simulink model "Control_model_10DOF_fin"  (R2016b)
settings: Solver=FixedStepAuto  StartTime=0.0  StopTime=10  FixedStep=0.0001  RelTol=1e-3
InitFcn:
  | Initialisation_ctr_10DOF_fin
values from neighbouring files (symbols this model uses):
  COM_Parameters = [-lpelvis/2;r2;0]    [Initialisation_ctr_10DOF_fin.m]
  DH_Parameters = [hfoot 0 ... (first row only)    [Initialisation_ctr_10DOF_fin.m]
  dTrunk = trunklbd(3)    [Initialisation_ctr_10DOF_fin.m]
  dxFootSM = dxFoot    [Initialisation_ctr_10DOF_fin.m]
  dxTrunk = 0.1    [Initialisation_ctr_10DOF_fin.m]
  Foot_Parameters = [0;-(lFoot/2-lHeel);0]    [Initialisation_ctr_10DOF_fin.m]
  HAA2HEE = [0; 0; 0.001]    [Initialisation_ctr_10DOF_fin.m]
  HEE2HFE = 0.5*[0.2; 0; 0]    [Initialisation_ctr_10DOF_fin.m]
  height_vrp = CoM_position(1)    [Initialisation_ctr_10DOF_fin.m]
  hTrunk = trunklbd(1)    [Initialisation_ctr_10DOF_fin.m]
  initial_CoM_position = R*CoM_position    [Initialisation_ctr_10DOF_fin.m]
  initial_CoM_velocity = [0;0;0]    [Initialisation_ctr_10DOF_fin.m]
  initial_left_foot = [0;0;-stance_width/2]    [Initialisation_ctr_10DOF_fin.m]
  initial_right_foot = [0;0;stance_width/2]    [Initialisation_ctr_10DOF_fin.m]
  initial_RorL = 0    [Initialisation_ctr_10DOF_fin.m]
  jointsinitial = [9;-15;6;0;0;6;-15;9]/180*pi    [Initialisation_ctr_10DOF_fin.m]
  K_DCM = 4.3*[1 0 0 ... (first row only)    [Initialisation_ctr_10DOF_fin.m]
  kD_left = mbody*[0.95 0 0 0 ... (first row only)    [Initialisation_ctr_10DOF_fin.m]
  kD_right = mbody*[0.12 0 0 0 ... (first row only)    [Initialisation_ctr_10DOF_fin.m]
  kI_left = mbody*[35 0 0 0 ... (first row only)    [Initialisation_ctr_10DOF_fin.m]
  kI_right = mbody*[38.2 0 0 0 ... (first row only)    [Initialisation_ctr_10DOF_fin.m]
  kP_left = mbody*[75 0 0 0 ... (first row only)    [Initialisation_ctr_10DOF_fin.m]
  kP_right = mbody*[5.6 0 0 0 ... (first row only)    [Initialisation_ctr_10DOF_fin.m]
  Lenght = [lShank;lThigh]    [Initialisation_ctr_10DOF_fin.m]
  lFootSM = lFoot    [Initialisation_ctr_10DOF_fin.m]
  lpelvis = wPelvis    [Initialisation_ctr_10DOF_fin.m]
  mass = mbody    (= 60)    [Initialisation_ctr_10DOF_fin.m]
  Masses = [mThigh; mShank; mTrunk]    [Initialisation_ctr_10DOF_fin.m]
  nb_step = 4    [Initialisation_ctr_10DOF_fin.m]
  nb_step_pattern = 20    [Initialisation_ctr_10DOF_fin.m]
  Pelvis_Parameters = [-lpelvis/2;hTrunk/2;0]    [Initialisation_ctr_10DOF_fin.m]
  stance_width = lpelvis    [Initialisation_ctr_10DOF_fin.m]
  stride_lenght = 0.50    (= 0.5)    [Initialisation_ctr_10DOF_fin.m]
  T_DS = time_DS    (= 0.4)    [Initialisation_ctr_10DOF_fin.m]
  T_IT = time_DS    (= 0.4)    [Initialisation_ctr_10DOF_fin.m]
  T_SS = time_swing    (= 1.6)    [Initialisation_ctr_10DOF_fin.m]
  time_DS = (time_stance-time_swing)/2    (= 0.4)    [Initialisation_ctr_10DOF_fin.m]
  time_stance = 60/100*time_stride    (= 2.4)    [Initialisation_ctr_10DOF_fin.m]
  time_step = time_stride/2    (= 2)    [Initialisation_ctr_10DOF_fin.m]
  time_swing = 40/100*time_stride    (= 1.6)    [Initialisation_ctr_10DOF_fin.m]
  validity_angle = [-20*pi/180 20*pi/180 ... (first row only)    [Initialisation_ctr_10DOF_fin.m]
  wTrunk = trunklbd(2)    [Initialisation_ctr_10DOF_fin.m]
  x4CoM = CoM_position(1)-XR4(1)    [Initialisation_ctr_10DOF_fin.m]
undefined symbols (not defined in the file or in its folder): dsegment, hFoot, l, lFoot, omega0_x, omega0_z, rho, wPelvis, X, Xp_x, Xp_z, Y, Z
undefined symbols (not defined in the file): k_grf, lShankSM, lThighSM, mShank, mThigh
libraries: nesl_utility x247, sm_lib x215, dspindex x12, FootPlacementLibrary x8, dspsigops x4, dspswit3 x1
(part 11 of 18)

== system Control_model_10DOF_fin/Control/Single_Support/Left Swing // Right Stance/Scope x8 ==
  Input : Inport
  Demux : Demux  Outputs=3
  Scope1 : Scope
  Scope2 : Scope
  Scope3 : Scope
  wires:
  Input/1 -> Demux/1
  Demux/2 -> Scope1/1
  Demux/3 -> Scope2/1
  Demux/1 -> Scope3/1

== system Control_model_10DOF_fin/Control/Single_Support/Left Swing // Right Stance/Stance leg position_initial ==
  position : Inport  PortDimensions=4
  velocity : Inport  Port=2  PortDimensions=4
  hip_trajectory : Inport  Port=3
  theta2 : Inport  Port=4
  Constant : Constant  Value=jointsinitial(1:4)
  Demux : Demux
  Mux : Mux
  PID right : Subsystem
  Scope x2 : Subsystem
  Sum1 : Sum  Inputs=-+|
  Terminator : Terminator
  Terminator1 : Terminator
  torques : Outport
  wires:
  PID right/1(torques_des) -> torques/1
  position/1 -> Scope x2/1(Input), Sum1/1
  Sum1/1 -> PID right/1(error)
  velocity/1 -> PID right/2(velocity)
  Constant/1 -> Demux/1
  Mux/1 -> Scope x2/2(Input1), Sum1/2
  Demux/1 -> Mux/1
  Demux/3 -> Mux/3
  hip_trajectory/1 -> Mux/4
  theta2/1 -> Mux/2
  Demux/2 -> Terminator/1
  Demux/4 -> Terminator1/1

== system Control_model_10DOF_fin/Control/Single_Support/Right Swing // Left Stance/Martijn Step adjustement ==
  FK_info : Inport
  R_or_L : Inport  Port=2
  Bus Selector : BusSelector  OutputSignals=XWcom,VWcom
  Constant1 : Constant  Value=time_swing
  Terminator : Terminator
  xCoM pred : Subsystem
  StepPos : Outport
  wires:
  Constant1/1 -> xCoM pred/1(T)
  R_or_L/1 -> xCoM pred/4(R_or_L)
  FK_info/1 -> Bus Selector/1
  Bus Selector/2 -> xCoM pred/3(Vcom)  "<VWcom>"
  Bus Selector/1 -> xCoM pred/2(Xcom)  "<XWcom>"
  xCoM pred/1(StepPos) -> StepPos/1
  xCoM pred/2(xCoMpred) -> Terminator/1

== system Control_model_10DOF_fin/Control/Single_Support/Right Swing // Left Stance/Right Swing leg control ==
  swing_state : Inport
  actual_joint_angle : Inport  Port=2
  FK_info : Inport  Port=3
  actual_joint_velocity : Inport  Port=4
  theta2 : Inport  Port=5
  Bus Selector : BusSelector  OutputSignals=TL4,TL1,TL0,TLR,TWL
  PID right : Subsystem
  Right : MATLAB Function  TreatAsAtomicUnit=on
  Saturation : Saturate  UpperLimit=validity_angle(1:4,2)  LowerLimit=validity_angle(1:4,1)
  Scope x2 : Subsystem
  Scope1 : Scope
  Scope2 : Scope
  Sum : Sum  Inputs=-+|
  Torques_des : Outport  OutDataTypeStr=double  Unit=N*m  PortDimensions=4
  wires:
  Right/1(desired_joint_angle) -> Saturation/1
  Sum/1 -> PID right/1(error)
  actual_joint_angle/1 -> Right/8(actual_joint_angle), Scope x2/1(Input), Sum/1
  FK_info/1 -> Bus Selector/1
  swing_state/1 -> Right/6(swing_state)
  actual_joint_velocity/1 -> PID right/2(velocity)
  PID right/1(torques_des) -> Torques_des/1
  Bus Selector/1 -> Right/1(TL4)  "<TL4>"
  Bus Selector/2 -> Right/2(TL1)  "<TL1>"
  Bus Selector/3 -> Right/3(TL0)  "<TL0>"
  Bus Selector/4 -> Right/4(TLR)  "<TLR>"
  Bus Selector/5 -> Right/5(TWL)  "<TWL>"
  Right/3(cas) -> Scope1/1
  Saturation/1 -> Sum/2, Scope x2/2(Input1)
  Right/2(ok) -> Scope2/1
  theta2/1 -> Right/7(desired_knee_angle)

== system Control_model_10DOF_fin/Control/Single_Support/Right Swing // Left Stance/Stance leg control ==
  DCM_position : Inport
  DCM_velocity : Inport  Port=2
  FK_info : Inport  Port=3
  Bus Selector : BusSelector  OutputSignals=XWcom,VWcom
  Bus Selector1 : BusSelector  OutputSignals=JLcom,TWL
  Bus Selector2 : BusSelector  OutputSignals=TWL
  Bus Selector3 : BusSelector  OutputSignals=XWcom
  DCM calcul : MATLAB Function  TreatAsAtomicUnit=on
  MATLAB Function : MATLAB Function  TreatAsAtomicUnit=on
  MATLAB Function1 : MATLAB Function  TreatAsAtomicUnit=on
  MATLAB Function2 : MATLAB Function  TreatAsAtomicUnit=on
  MATLAB Function5 : MATLAB Function  TreatAsAtomicUnit=on
  Terminator : Terminator
  Terminator1 : Terminator
  VRP based DCM tracking control : MATLAB Function  TreatAsAtomicUnit=on
  Torques_des : Outport  OutDataTypeStr=double  Unit=N*m
  Force_des : Outport  Port=2
  r_vrp : Outport  Port=3
  r_extrapolated_CoM : Outport  Port=4
  wires:
  DCM_position/1 -> VRP based DCM tracking control/3(DCM_position)
  DCM_velocity/1 -> VRP based DCM tracking control/2(DCM_velocity)
  Bus Selector/1 -> DCM calcul/1(CoM_position)  "<XWcom>"
  DCM calcul/1(r_DCM) -> VRP based DCM tracking control/1(r_DCM), r_extrapolated_CoM/1
  MATLAB Function/1(Force_des) -> MATLAB Function2/1(Force_des)
  MATLAB Function2/1(Torques_des) -> Torques_des/1
  Bus Selector/2 -> DCM calcul/2(CoM_velocity)  "<VWcom>"
  Bus Selector1/1 -> MATLAB Function2/2(JcomL)  "<JLcom>"
  MATLAB Function5/1(new_vrp_W) -> MATLAB Function/1(r_vrp)
  VRP based DCM tracking control/1(r_vrp) -> r_vrp/1, MATLAB Function1/1(r_vrp), MATLAB Function5/1(r_vrp_W)
  Bus Selector2/1 -> MATLAB Function1/3(TWL), MATLAB Function5/2(TWL)  "<TWL>"
  Bus Selector3/1 -> MATLAB Function1/2(r_CoM), MATLAB Function/2(r_CoM)  "<XWcom>"
  Bus Selector1/2 -> MATLAB Function2/3(TWL)  "<TWL>"
  FK_info/1 -> Bus Selector1/1, Bus Selector3/1, Bus Selector2/1, Bus Selector/1
  MATLAB Function1/1(Force_des) -> Force_des/1
  MATLAB Function5/2(outside) -> Terminator/1
  MATLAB Function5/3(cas) -> Terminator1/1

== system Control_model_10DOF_fin/Control/Single_Support/Right Swing // Left Stance/Stance leg position_initial1 ==
  position : Inport  PortDimensions=4
  velocity : Inport  Port=2  PortDimensions=4
  hip_trajectory : Inport  Port=3
  theta7 : Inport  Port=4
  Constant : Constant  Value=jointsinitial(5:8)
  Demux1 : Demux
  Mux1 : Mux
  PID left : Subsystem
  Scope : Scope
  Sum1 : Sum  Inputs=-+|
  Terminator : Terminator
  Terminator1 : Terminator
  torques : Outport
  wires:
  position/1 -> Sum1/1
  Sum1/1 -> Scope/1, PID left/1(error)
  velocity/1 -> PID left/2(velocity)
  PID left/1(torques_des) -> torques/1
  Constant/1 -> Demux1/1
  Mux1/1 -> Sum1/2
  Demux1/2 -> Mux1/2
  Demux1/4 -> Mux1/4
  hip_trajectory/1 -> Mux1/1
  theta7/1 -> Mux1/3
  Demux1/1 -> Terminator/1
  Demux1/3 -> Terminator1/1

== system Control_model_10DOF_fin/Control/Stance_position/Stance control/PID left ==
  error : Inport  PortDimensions=4
  velocity : Inport  Port=2
  Filter : Integrator  Commented=on  DisableCoverage=on
  Gain : Gain  Commented=on  Gain=100
  Integrator : Integrator
  Product{,1..3} (4 alike) : Product  Multiplication=Matrix(*)
  Sum : Sum  Inputs=++-
  Sum1 : Sum  Commented=on  Inputs=|+-
  kD : Constant  Value=kD_left
  kI : Constant  Value=kI_left
  kP : Constant  Value=kP_left
  torques_des : Outport  PortDimensions=4  InitialOutput=0
  wires:
  Sum/1 -> torques_des/1
  Gain/1 -> Filter/1
  Sum1/1 -> Gain/1
  Product/1 -> Sum/1
  error/1 -> Product2/2, Product1/2, Product/2
  Product1/1 -> Sum1/1
  kP/1 -> Product/1
  Filter/1 -> Sum1/2
  Integrator/1 -> Sum/2
  Product2/1 -> Integrator/1
  kI/1 -> Product2/1
  kD/1 -> Product3/1, Product1/1
  velocity/1 -> Product3/2
  Product3/1 -> Sum/3

== system Control_model_10DOF_fin/Control/Stance_position/Stance control/PID right ==
  error : Inport  PortDimensions=4
  velocity : Inport  Port=2
  Filter : Integrator  Commented=on  DisableCoverage=on
  Gain : Gain  Commented=on  Gain=100
  Integrator : Integrator
  Product{,1..3} (4 alike) : Product  Multiplication=Matrix(*)
  Sum : Sum  Inputs=++-
  Sum1 : Sum  Commented=on  Inputs=|+-
  kD : Constant  Value=kD_right
  kI : Constant  Value=kI_right
  kP : Constant  Value=kP_right
  torques_des : Outport  PortDimensions=4  InitialOutput=0
  wires:
  Sum/1 -> torques_des/1
  Gain/1 -> Filter/1
  Sum1/1 -> Gain/1
  Product/1 -> Sum/1
  error/1 -> Product2/2, Product1/2, Product/2
  Product1/1 -> Sum1/1
  kP/1 -> Product/1
  Filter/1 -> Sum1/2
  Integrator/1 -> Sum/2
  Product2/1 -> Integrator/1
  kI/1 -> Product2/1
  kD/1 -> Product3/1, Product1/1
  velocity/1 -> Product3/2
  Product3/1 -> Sum/3

== system Control_model_10DOF_fin/Control/Stance_position/Stance control/scope system ==
  input : Inport
  input2 : Inport  Port=2
  Demux : Demux  Outputs=8
  Demux1 : Demux  Outputs=8
  Gain1 : Gain  Gain=180/pi
  Gain3 : Gain  Gain=180/pi
  Scope{,1..7} (8 alike) : Scope  NumInputPorts=2
  wires:
  input/1 -> Gain3/1
  Demux/1 -> Scope/1
  Demux/2 -> Scope1/1
  Gain3/1 -> Demux/1
  input2/1 -> Gain1/1
  Gain1/1 -> Demux1/1
  Demux1/1 -> Scope/2
  Demux1/2 -> Scope1/2
  Demux/3 -> Scope2/1
  Demux1/3 -> Scope2/2
  Demux/4 -> Scope3/1
  Demux1/4 -> Scope3/2
  Demux/5 -> Scope4/1
  Demux1/5 -> Scope4/2
  Demux/6 -> Scope5/1
  Demux1/6 -> Scope5/2
  Demux/7 -> Scope6/1
  Demux1/7 -> Scope6/2
  Demux/8 -> Scope7/1
  Demux1/8 -> Scope7/2

== system Control_model_10DOF_fin/Control/Stance_position/Stance control/scope system1 ==
  input : Inport
  Demux : Demux  Outputs=8
  Gain3 : Gain  Gain=180/pi
  Scope{,1..7} (8 alike) : Scope
  wires:
  input/1 -> Gain3/1
  Demux/1 -> Scope/1
  Demux/2 -> Scope1/1
  Demux/3 -> Scope2/1
  Demux/5 -> Scope4/1
  Demux/7 -> Scope6/1
  Demux/8 -> Scope7/1
  Demux/4 -> Scope3/1
  Demux/6 -> Scope5/1
  Gain3/1 -> Demux/1

== system Control_model_10DOF_fin/Time//State Machine/Hip_timer/SS/First_part ==
  Action Port : ActionPort  ActionType=then
  Constant : Constant  Value=0
  time_Hip : Outport
  wires:
  Constant/1 -> time_Hip/1

== system Control_model_10DOF_fin/Time//State Machine/Hip_timer/SS/Second_part ==
  time_swing : Inport
  Action Port : ActionPort  ActionType=else
  Constant : Constant  Value=time_swing/2
  Sum1 : Sum  Inputs=|+-
  time_Hip : Outport
  wires:
  Sum1/1 -> time_Hip/1
  Constant/1 -> Sum1/2
  time_swing/1 -> Sum1/1

== system Control_model_10DOF_fin/Trajectory generator/DCM trajectory/DS/Scope x8 ==
  Input : Inport
  Demux : Demux  Outputs=3
  Scope1 : Scope
  Scope2 : Scope
  Scope3 : Scope
  wires:
  Input/1 -> Demux/1
  Demux/2 -> Scope1/1
  Demux/3 -> Scope2/1
  Demux/1 -> Scope3/1

== system Control_model_10DOF_fin/Trajectory generator/DCM trajectory/Initial_Transfert/DCM_estimate_fin ==
  r_vrp : Inport
  r_DCM : Inport  Port=2
  time : Inport  Port=3
  DCM trajectory generator : MATLAB Function  TreatAsAtomicUnit=on
  DCM_position : Outport
  DCM_velocity : Outport  Port=2
  wires:
  r_vrp/1 -> DCM trajectory generator/1(r_vrp)
  r_DCM/1 -> DCM trajectory generator/2(r_DCM)
  time/1 -> DCM trajectory generator/3(time)
  DCM trajectory generator/1(DCM_position) -> DCM_position/1
  DCM trajectory generator/2(DCM_velocity) -> DCM_velocity/1

== system Control_model_10DOF_fin/Trajectory generator/Enabled and Triggered Subsystem 1/Feet Pattern generator/initial position ==
  Constant : Constant  Value=initial_RorL
  If first right swing : If  IfExpression=u1 ==1
  Merge1 : Merge
  Merge2 : Merge
  initial position : Subsystem  TreatAsAtomicUnit=on
  initial position1 : Subsystem  TreatAsAtomicUnit=on
  initial_swing_foot : Outport
  initial_stance_foot : Outport  Port=2
  wires:
  If first right swing/1 -> initial position/Action
  If first right swing/2 -> initial position1/Action
  initial position/1(initial_swing_foot) -> Merge1/1
  initial position/2(initial_stance_foot) -> Merge2/1
  Merge1/1 -> initial_swing_foot/1
  Merge2/1 -> initial_stance_foot/1
  Constant/1 -> If first right swing/1
  initial position1/1(initial_swing_foot) -> Merge1/2
  initial position1/2(initial_stance_foot) -> Merge2/2

== system Control_model_10DOF_fin/Trajectory generator/Enabled and Triggered Subsystem 1/initial position/initial position ==
  Action Port : ActionPort  ActionType=then
  Constant : Constant  Value=initial_right_foot
  Constant1 : Constant  Value=initial_left_foot
  initial_swing_foot : Outport
  initial_stance_foot : Outport  Port=2
  wires:
  Constant/1 -> initial_swing_foot/1
  Constant1/1 -> initial_stance_foot/1

== system Control_model_10DOF_fin/Trajectory generator/Enabled and Triggered Subsystem 1/initial position/initial position1 ==
  Action Port : ActionPort  ActionType=else
  Constant : Constant  Value=initial_left_foot
  Constant1 : Constant  Value=initial_right_foot
  initial_swing_foot : Outport
  initial_stance_foot : Outport  Port=2
  wires:
  Constant/1 -> initial_swing_foot/1
  Constant1/1 -> initial_stance_foot/1

== system Control_model_10DOF_fin/Trajectory generator/Enabled and Triggered Subsystem 1/initial position1/Left ==
  Right_foot : Inport
  Left_foot : Inport  Port=2
  Action Port : ActionPort  ActionType=else
  MATLAB Function : MATLAB Function  TreatAsAtomicUnit=on
  MATLAB Function1 : MATLAB Function  TreatAsAtomicUnit=on
  initial_swing_foot : Outport
  initial_stance_foot : Outport  Port=2
  wires:
  Right_foot/1 -> MATLAB Function1/1(T)
  MATLAB Function1/1(X) -> initial_stance_foot/1
  Left_foot/1 -> MATLAB Function/1(T)
  MATLAB Function/1(X) -> initial_swing_foot/1

== system Control_model_10DOF_fin/Trajectory generator/Enabled and Triggered Subsystem 1/initial position1/Right ==
  Right_foot : Inport
  Left_foot : Inport  Port=2
  Action Port : ActionPort  ActionType=then
  MATLAB Function : MATLAB Function  TreatAsAtomicUnit=on
  MATLAB Function1 : MATLAB Function  TreatAsAtomicUnit=on
  initial_swing_foot : Outport
  initial_stance_foot : Outport  Port=2
  wires:
  Right_foot/1 -> MATLAB Function/1(T)
  MATLAB Function/1(X) -> initial_swing_foot/1
  Left_foot/1 -> MATLAB Function1/1(T)
  MATLAB Function1/1(X) -> initial_stance_foot/1

== system Control_model_10DOF_fin/Trajectory generator/Enabled and Triggered Subsystem 1/initial position2/Left ==
  Right_foot : Inport
  Left_foot : Inport  Port=2
  Action Port : ActionPort  ActionType=else
  MATLAB Function : MATLAB Function  TreatAsAtomicUnit=on
  MATLAB Function1 : MATLAB Function  TreatAsAtomicUnit=on
  initial_swing_foot : Outport
  initial_stance_foot : Outport  Port=2
  wires:
  Right_foot/1 -> MATLAB Function1/1(T)
  MATLAB Function1/1(X) -> initial_stance_foot/1
  Left_foot/1 -> MATLAB Function/1(T)
  MATLAB Function/1(X) -> initial_swing_foot/1

== system Control_model_10DOF_fin/Trajectory generator/Enabled and Triggered Subsystem 1/initial position2/Right ==
  Right_foot : Inport
  Left_foot : Inport  Port=2
  Action Port : ActionPort  ActionType=then
  MATLAB Function : MATLAB Function  TreatAsAtomicUnit=on
  MATLAB Function1 : MATLAB Function  TreatAsAtomicUnit=on
  initial_swing_foot : Outport
  initial_stance_foot : Outport  Port=2
  wires:
  Right_foot/1 -> MATLAB Function/1(T)
  MATLAB Function/1(X) -> initial_swing_foot/1
  Left_foot/1 -> MATLAB Function1/1(T)
  MATLAB Function1/1(X) -> initial_stance_foot/1

== system Control_model_10DOF_fin/Trajectory generator/Enabled and Triggered Subsystem 1/selector/1 ==
  In1 : Inport
  Constant : Constant  Value=2
  Constant1 : Constant  Value=3
  Constant2 : Constant
  Product : Product
  Sum : Sum  Inputs=|++
  Sum1 : Sum  Inputs=|++
  Out1 : Outport
  wires:
  Constant1/1 -> Product/1
  Constant2/1 -> Sum1/2
  Sum1/1 -> Out1/1
  Sum/1 -> Product/2
  Constant/1 -> Sum/2
  In1/1 -> Sum/1
  Product/1 -> Sum1/1

== system Control_model_10DOF_fin/Trajectory generator/Enabled and Triggered Subsystem 1/selector/2 ==
  In1 : Inport
  Constant : Constant  Value=2
  Constant1 : Constant  Value=3
  Constant2 : Constant  Value=2
  Product : Product
  Sum : Sum  Inputs=|++
  Sum1 : Sum  Inputs=|++
  Out1 : Outport
  wires:
  Constant1/1 -> Product/1
  Constant2/1 -> Sum1/2
  Sum1/1 -> Out1/1
  Sum/1 -> Product/2
  Constant/1 -> Sum/2
  In1/1 -> Sum/1
  Product/1 -> Sum1/1

== system Control_model_10DOF_fin/Trajectory generator/Enabled and Triggered Subsystem 1/selector/3 ==
  In1 : Inport
  Constant : Constant  Value=2
  Constant1 : Constant  Value=3
  Constant2 : Constant  Value=3
  Product : Product
  Sum : Sum  Inputs=|++
  Sum1 : Sum  Inputs=|++
  Out1 : Outport
  wires:
  Constant1/1 -> Product/1
  Constant2/1 -> Sum1/2
  Sum1/1 -> Out1/1
  Sum/1 -> Product/2
  Constant/1 -> Sum/2
  In1/1 -> Sum/1
  Product/1 -> Sum1/1

== system Control_model_10DOF_fin/Trajectory generator/Enabled and Triggered Subsystem 1/selector1/1 ==
  In1 : Inport
  Constant : Constant
  Constant1 : Constant  Value=3
  Constant2 : Constant
  Product : Product
  Sum : Sum  Inputs=|++
  Sum1 : Sum  Inputs=|++
  Out1 : Outport
  wires:
  Constant1/1 -> Product/1
  Constant2/1 -> Sum1/2
  Sum1/1 -> Out1/1
  Sum/1 -> Product/2
  Constant/1 -> Sum/2
  In1/1 -> Sum/1
  Product/1 -> Sum1/1

== system Control_model_10DOF_fin/Trajectory generator/Enabled and Triggered Subsystem 1/selector1/2 ==
  In1 : Inport
  Constant : Constant
  Constant1 : Constant  Value=3
  Constant2 : Constant  Value=2
  Product : Product
  Sum : Sum  Inputs=|++
  Sum1 : Sum  Inputs=|++
  Out1 : Outport
  wires:
  Constant1/1 -> Product/1
  Constant2/1 -> Sum1/2
  Sum1/1 -> Out1/1
  Sum/1 -> Product/2
  Constant/1 -> Sum/2
  In1/1 -> Sum/1
  Product/1 -> Sum1/1

== system Control_model_10DOF_fin/Trajectory generator/Enabled and Triggered Subsystem 1/selector1/3 ==
  In1 : Inport
  Constant : Constant
  Constant1 : Constant  Value=3
  Constant2 : Constant  Value=3
  Product : Product
  Sum : Sum  Inputs=|++
  Sum1 : Sum  Inputs=|++
  Out1 : Outport
  wires:
  Constant1/1 -> Product/1
  Constant2/1 -> Sum1/2
  Sum1/1 -> Out1/1
  Sum/1 -> Product/2
  Constant/1 -> Sum/2
  In1/1 -> Sum/1
  Product/1 -> Sum1/1

== system Control_model_10DOF_fin/Trajectory generator/Enabled and Triggered Subsystem 1/selector2/1 ==
  In1 : Inport
  Constant : Constant  Value=0
  Constant1 : Constant  Value=3
  Constant2 : Constant
  Product : Product
  Sum : Sum  Inputs=|++
  Sum1 : Sum  Inputs=|++
  Out1 : Outport
  wires:
  Constant1/1 -> Product/1
  Constant2/1 -> Sum1/2
  Sum1/1 -> Out1/1
  Sum/1 -> Product/2
  Constant/1 -> Sum/2
  In1/1 -> Sum/1
  Product/1 -> Sum1/1

== system Control_model_10DOF_fin/Trajectory generator/Enabled and Triggered Subsystem 1/selector2/2 ==
  In1 : Inport
  Constant : Constant  Value=0
  Constant1 : Constant  Value=3
  Constant2 : Constant  Value=2
  Product : Product
  Sum : Sum  Inputs=|++
  Sum1 : Sum  Inputs=|++
  Out1 : Outport
  wires:
  Constant1/1 -> Product/1
  Constant2/1 -> Sum1/2
  Sum1/1 -> Out1/1
  Sum/1 -> Product/2
  Constant/1 -> Sum/2
  In1/1 -> Sum/1
  Product/1 -> Sum1/1

== system Control_model_10DOF_fin/Trajectory generator/Enabled and Triggered Subsystem 1/selector2/3 ==
  In1 : Inport
  Constant : Constant  Value=0
  Constant1 : Constant  Value=3
  Constant2 : Constant  Value=3
  Product : Product
  Sum : Sum  Inputs=|++
  Sum1 : Sum  Inputs=|++
  Out1 : Outport
  wires:
  Constant1/1 -> Product/1
  Constant2/1 -> Sum1/2
  Sum1/1 -> Out1/1
  Sum/1 -> Product/2
  Constant/1 -> Sum/2
  In1/1 -> Sum/1
  Product/1 -> Sum1/1

== system Control_model_10DOF_fin/Trajectory generator/Enabled and Triggered Subsystem 1/selector3/1 ==
  In1 : Inport
  Constant : Constant  Value=3
  Constant1 : Constant  Value=3
  Constant2 : Constant
  Product : Product
  Sum : Sum  Inputs=|++
  Sum1 : Sum  Inputs=|++
  Out1 : Outport
  wires:
  Constant1/1 -> Product/1
  Constant2/1 -> Sum1/2
  Sum1/1 -> Out1/1
  Sum/1 -> Product/2
  Constant/1 -> Sum/2
  In1/1 -> Sum/1
  Product/1 -> Sum1/1

== system Control_model_10DOF_fin/Trajectory generator/Enabled and Triggered Subsystem 1/selector3/2 ==
  In1 : Inport
  Constant : Constant  Value=3
  Constant1 : Constant  Value=3
  Constant2 : Constant  Value=2
  Product : Product
  Sum : Sum  Inputs=|++
  Sum1 : Sum  Inputs=|++
  Out1 : Outport
  wires:
  Constant1/1 -> Product/1
  Constant2/1 -> Sum1/2
  Sum1/1 -> Out1/1
  Sum/1 -> Product/2
  Constant/1 -> Sum/2
  In1/1 -> Sum/1
  Product/1 -> Sum1/1

== system Control_model_10DOF_fin/Trajectory generator/Enabled and Triggered Subsystem 1/selector3/3 ==
  In1 : Inport
  Constant : Constant  Value=3
  Constant1 : Constant  Value=3
  Constant2 : Constant  Value=3
  Product : Product
  Sum : Sum  Inputs=|++
  Sum1 : Sum  Inputs=|++
  Out1 : Outport
  wires:
  Constant1/1 -> Product/1
  Constant2/1 -> Sum1/2
  Sum1/1 -> Out1/1
  Sum/1 -> Product/2
  Constant/1 -> Sum/2
  In1/1 -> Sum/1
  Product/1 -> Sum1/1

== system Control_model_10DOF_fin/Trajectory generator/Hip trajectory2/SS/Subsystem1 ==
  Action Port : ActionPort  ActionType=else
  Constant : Constant  Value=0
  hip_trajectory : Outport
  wires:
  Constant/1 -> hip_trajectory/1

== system Control_model_10DOF_fin/Trajectory generator/Hip trajectory2/SS/Subsystem2 ==
  time_Hip : Inport
  Action Port : ActionPort  ActionType=then
  If first part of swing : If  IfExpression=u1 ==0
  Merge2 : Merge
  Subsystem : Subsystem
  Subsystem1 : Subsystem
  hip_trajectory : Outport
  wires:
  time_Hip/1 -> Subsystem/1(time_Hip), If first part of swing/1
  Merge2/1 -> hip_trajectory/1
  If first part of swing/1 -> Subsystem1/Action
  Subsystem1/1(hip_trajectory) -> Merge2/1
  If first part of swing/2 -> Subsystem/Action
  Subsystem/1(hip_trajectory) -> Merge2/2

== system Control_model_10DOF_fin/Trajectory generator/knee trajectory/DS/Left transfer ==
  time_swing : Inport  OutDataTypeStr=double  Unit=s  PortDimensions=1
  joint_angle : Inport  Port=2
  Action Port : ActionPort  ActionType=then
  Constant : Constant  Value=-15*pi/180
  Mux : Mux  Inputs=2
  Swing leg trajectory1 : MATLAB Function  TreatAsAtomicUnit=on
  theta7 : Selector  InputPortWidth=8  IndexOptions=Index vector (dialog)  Indices=[7]  OutputSizes=1
  knee_trajectory : Outport
  wires:
  Mux/1 -> knee_trajectory/1
  Swing leg trajectory1/1(knee_angle_des) -> Mux/2
  joint_angle/1 -> theta7/1
  time_swing/1 -> Swing leg trajectory1/1(current_time)
  Constant/1 -> Mux/1
  theta7/1 -> Swing leg trajectory1/2(knee_angle_ini)

== system Control_model_10DOF_fin/Trajectory generator/knee trajectory/DS/Right transfer ==
  time_swing : Inport  OutDataTypeStr=double  Unit=s  PortDimensions=1
  joint_angle : Inport  Port=2
  Action Port : ActionPort  ActionType=else
  Constant : Constant  Value=-15*pi/180
  Mux : Mux  Inputs=2
  Swing leg trajectory1 : MATLAB Function  TreatAsAtomicUnit=on
  theta2 : Selector  InputPortWidth=8  IndexOptions=Index vector (dialog)  Indices=[2]  OutputSizes=1
  knee_trajectory : Outport
  wires:
  Mux/1 -> knee_trajectory/1
  joint_angle/1 -> theta2/1
  time_swing/1 -> Swing leg trajectory1/1(current_time)
  Swing leg trajectory1/1(knee_angle_des) -> Mux/1
  Constant/1 -> Mux/2
  theta2/1 -> Swing leg trajectory1/2(knee_angle_ini)

== system Control_model_10DOF_fin/Trajectory generator/knee trajectory/SS/Left swing  ==
  time_swing : Inport  OutDataTypeStr=double  Unit=s  PortDimensions=1
  joint_angle : Inport  Port=2
  Action Port : ActionPort  ActionType=then
  Constant : Constant  Value=time_swing/2
  If first part of swing : If  IfExpression=u1 <= half_time_swing
  Merge2 : Merge
  Mux : Mux  Inputs=2
  Sum1 : Sum  Inputs=|+-
  Swing leg trajectory1 : MATLAB Function  TreatAsAtomicUnit=on
  knee trajectory : Subsystem  TreatAsAtomicUnit=on
  knee trajectory1 : Subsystem  TreatAsAtomicUnit=on
  theta2 : Selector  InputPortWidth=8  IndexOptions=Index vector (dialog)  Indices=[2]  OutputSizes=1
  theta7 : Selector  InputPortWidth=8  IndexOptions=Index vector (dialog)  Indices=[7]  OutputSizes=1
  knee_trajectory : Outport
  wires:
  Mux/1 -> knee_trajectory/1
  If first part of swing/1 -> knee trajectory/Action
  If first part of swing/2 -> knee trajectory1/Action
  knee trajectory/1(knee_angle_des) -> Merge2/1
  knee trajectory1/1(knee_angle_des) -> Merge2/2
  knee trajectory/2(knee_angle_des2) -> knee trajectory1/2(knee_angle_ini)
  Merge2/1 -> Mux/2
  Sum1/1 -> knee trajectory1/1(current_time)
  Constant/1 -> Sum1/2
  time_swing/1 -> Sum1/1, knee trajectory/1(current_time), Swing leg trajectory1/1(current_time), If first part of swing/1
  joint_angle/1 -> theta2/1, theta7/1
  Swing leg trajectory1/1(knee_angle_des) -> Mux/1
  theta7/1 -> knee trajectory/2(knee_angle_ini)
  theta2/1 -> Swing leg trajectory1/2(knee_angle_ini)

== system Control_model_10DOF_fin/Trajectory generator/knee trajectory/SS/Right swing ==
  time_swing : Inport  OutDataTypeStr=double  Unit=s  PortDimensions=1
  joint_angle : Inport  Port=2
  Action Port : ActionPort  ActionType=else
  Constant : Constant  Value=time_swing/2
  If first part of swing : If  IfExpression=u1 <= half_time_swing
  Merge2 : Merge
  Mux : Mux  Inputs=2
  Scope : Scope
  Sum1 : Sum  Inputs=|+-
  Swing leg trajectory1 : MATLAB Function  TreatAsAtomicUnit=on
  knee trajectory : Subsystem  TreatAsAtomicUnit=on
  knee trajectory1 : Subsystem  TreatAsAtomicUnit=on
  theta2 : Selector  InputPortWidth=8  IndexOptions=Index vector (dialog)  Indices=[2]  OutputSizes=1
  theta7 : Selector  InputPortWidth=8  IndexOptions=Index vector (dialog)  Indices=[7]  OutputSizes=1
  knee_trajectory : Outport
  wires:
  Mux/1 -> knee_trajectory/1
  If first part of swing/1 -> knee trajectory/Action
  If first part of swing/2 -> knee trajectory1/Action
  knee trajectory/1(knee_angle_des) -> Merge2/1
  knee trajectory1/1(knee_angle_des) -> Merge2/2
  knee trajectory/2(knee_angle_des2) -> knee trajectory1/2(knee_angle_ini)
  Sum1/1 -> knee trajectory1/1(current_time)
  Constant/1 -> Sum1/2
  joint_angle/1 -> theta2/1, theta7/1
  Merge2/1 -> Mux/1
  Swing leg trajectory1/1(knee_angle_des) -> Mux/2
  time_swing/1 -> Scope/1, Swing leg trajectory1/1(current_time), Sum1/1, knee trajectory/1(current_time), If first part of swing/1
  theta2/1 -> knee trajectory/2(knee_angle_ini)
  theta7/1 -> Swing leg trajectory1/2(knee_angle_ini)

== system Control_model_10DOF_fin/Control/Double_Support/Left stance phase1/Stance leg position_initial/PID right ==
  error : Inport  PortDimensions=4
  velocity : Inport  Port=2
  Integrator : Integrator
  Product : Product  Multiplication=Matrix(*)
  Product2 : Product  Multiplication=Matrix(*)
  Product3 : Product  Multiplication=Matrix(*)
  Sum : Sum  Inputs=++-
  kD : Constant  Value=kD_right
  kI : Constant  Value=kI_right
  kP : Constant  Value=kP_right
  torques_des : Outport  PortDimensions=4  InitialOutput=0
  wires:
  Sum/1 -> torques_des/1
  Product/1 -> Sum/1
  error/1 -> Product2/2, Product/2
  kP/1 -> Product/1
  Integrator/1 -> Sum/2
  Product2/1 -> Integrator/1
  kI/1 -> Product2/1
  kD/1 -> Product3/1
  velocity/1 -> Product3/2
  Product3/1 -> Sum/3

== system Control_model_10DOF_fin/Control/Double_Support/Left stance phase1/Stance leg position_initial/Scope x1 ==
  Input : Inport
  Demux : Demux
  Scop e1 : Scope
  Scope1 : Scope
  Scope2 : Scope
  Scope3 : Scope
  wires:
  Input/1 -> Demux/1
  Demux/2 -> Scop e1/1
  Demux/3 -> Scope2/1
  Demux/1 -> Scope3/1
  Demux/4 -> Scope1/1

== system Control_model_10DOF_fin/Control/Double_Support/Left stance phase1/Stance leg position_initial1/PID left ==
  error : Inport  PortDimensions=4
  velocity : Inport  Port=2
  Integrator : Integrator
  Product : Product  Multiplication=Matrix(*)
  Product2 : Product  Multiplication=Matrix(*)
  Product3 : Product  Multiplication=Matrix(*)
  Sum : Sum  Inputs=++-
  kD : Constant  Value=kD_left
  kI : Constant  Value=kI_left
  kP : Constant  Value=kP_left
  torques_des : Outport  PortDimensions=4  InitialOutput=0
  wires:
  Sum/1 -> torques_des/1
  Product/1 -> Sum/1
  error/1 -> Product2/2, Product/2
  kP/1 -> Product/1
  Integrator/1 -> Sum/2
  Product2/1 -> Integrator/1
  kI/1 -> Product2/1
  kD/1 -> Product3/1
  velocity/1 -> Product3/2
  Product3/1 -> Sum/3

== system Control_model_10DOF_fin/Control/Double_Support/Left stance phase1/Stance leg position_initial1/Scope x2 ==
  Input : Inport
  Input1 : Inport  Port=2
  Demux : Demux
  Demux1 : Demux
  Scope{,1..3} (4 alike) : Scope  NumInputPorts=2
  wires:
  Input/1 -> Demux/1
  Demux/2 -> Scope1/1
  Demux/3 -> Scope2/1
  Demux/1 -> Scope3/1
  Input1/1 -> Demux1/1
  Demux1/1 -> Scope3/2
  Demux1/2 -> Scope1/2
  Demux1/3 -> Scope2/2
  Demux1/4 -> Scope/2
  Demux/4 -> Scope/1

== system Control_model_10DOF_fin/Control/Double_Support/Right stance phase/Stance leg position_initial/PID right ==
  error : Inport  PortDimensions=4
  velocity : Inport  Port=2
  Integrator : Integrator
  Product : Product  Multiplication=Matrix(*)
  Product2 : Product  Multiplication=Matrix(*)
  Product3 : Product  Multiplication=Matrix(*)
  Sum : Sum  Inputs=++-
  kD : Constant  Value=kD_right
  kI : Constant  Value=kI_right
  kP : Constant  Value=kP_right
  torques_des : Outport  PortDimensions=4  InitialOutput=0
  wires:
  Sum/1 -> torques_des/1
  Product/1 -> Sum/1
  error/1 -> Product2/2, Product/2
  kP/1 -> Product/1
  Integrator/1 -> Sum/2
  Product2/1 -> Integrator/1
  kI/1 -> Product2/1
  kD/1 -> Product3/1
  velocity/1 -> Product3/2
  Product3/1 -> Sum/3

== system Control_model_10DOF_fin/Control/Double_Support/Right stance phase/Stance leg position_initial/Scope x2 ==
  Input : Inport
  Input1 : Inport  Port=2
  Demux : Demux
  Demux1 : Demux
  Scope{,1..3} (4 alike) : Scope  NumInputPorts=2
  wires:
  Input/1 -> Demux/1
  Demux/2 -> Scope1/1
  Demux/3 -> Scope2/1
  Demux/1 -> Scope3/1
  Input1/1 -> Demux1/1
  Demux1/1 -> Scope3/2
  Demux1/2 -> Scope1/2
  Demux1/3 -> Scope2/2
  Demux1/4 -> Scope/2
  Demux/4 -> Scope/1

== system Control_model_10DOF_fin/Control/Double_Support/Right stance phase/Stance leg position_initial1/PID left ==
  error : Inport  PortDimensions=4
  velocity : Inport  Port=2
  Integrator : Integrator
  Product : Product  Multiplication=Matrix(*)
  Product2 : Product  Multiplication=Matrix(*)
  Product3 : Product  Multiplication=Matrix(*)
  Sum : Sum  Inputs=++-
  kD : Constant  Value=kD_left
  kI : Constant  Value=kI_left
  kP : Constant  Value=kP_left
  torques_des : Outport  PortDimensions=4  InitialOutput=0
  wires:
  Sum/1 -> torques_des/1
  Product/1 -> Sum/1
  error/1 -> Product2/2, Product/2
  kP/1 -> Product/1
  Integrator/1 -> Sum/2
  Product2/1 -> Integrator/1
  kI/1 -> Product2/1
  kD/1 -> Product3/1
  velocity/1 -> Product3/2
  Product3/1 -> Sum/3

== system Control_model_10DOF_fin/Control/Double_Support/Right stance phase/Stance leg position_initial1/Scope x2 ==
  Input : Inport
  Input1 : Inport  Port=2
  Demux : Demux
  Demux1 : Demux
  Scope{,1..3} (4 alike) : Scope  NumInputPorts=2
  wires:
  Input/1 -> Demux/1
  Demux/2 -> Scope1/1
  Demux/3 -> Scope2/1
  Demux/1 -> Scope3/1
  Input1/1 -> Demux1/1
  Demux1/1 -> Scope3/2
  Demux1/2 -> Scope1/2
  Demux1/3 -> Scope2/2
  Demux1/4 -> Scope/2
  Demux/4 -> Scope/1

== system Control_model_10DOF_fin/Control/Finish_Swing_Phase/Left Swing // Right Stance/Left Swing leg control/PID left ==
  error : Inport  PortDimensions=4
  velocity : Inport  Port=2
  Integrator : Integrator
  Product : Product  Multiplication=Matrix(*)
  Product2 : Product  Multiplication=Matrix(*)
  Product3 : Product  Multiplication=Matrix(*)
  Sum : Sum  Inputs=++-
  kD : Constant  Value=kD_left
  kI : Constant  Value=kI_left
  kP : Constant  Value=kP_left
  torques_des : Outport  PortDimensions=4  InitialOutput=0
  wires:
  Sum/1 -> torques_des/1
  Product/1 -> Sum/1
  error/1 -> Product2/2, Product/2
  kP/1 -> Product/1
  Integrator/1 -> Sum/2
  Product2/1 -> Integrator/1
  kI/1 -> Product2/1
  kD/1 -> Product3/1
  velocity/1 -> Product3/2
  Product3/1 -> Sum/3

== system Control_model_10DOF_fin/Control/Finish_Swing_Phase/Left Swing // Right Stance/Left Swing leg control/Scope x1 ==
  Input : Inport
  Demux : Demux  Outputs=3
  Scope1 : Scope
  Scope2 : Scope
  Scope3 : Scope
  wires:
  Input/1 -> Demux/1
  Demux/2 -> Scope1/1
  Demux/3 -> Scope2/1
  Demux/1 -> Scope3/1

== system Control_model_10DOF_fin/Control/Finish_Swing_Phase/Left Swing // Right Stance/Left Swing leg control/Scope x2 ==
  Input : Inport
  Input1 : Inport  Port=2
  Demux : Demux
  Demux1 : Demux
  Scope{,1..3} (4 alike) : Scope  NumInputPorts=2
  wires:
  Input/1 -> Demux/1
  Demux/2 -> Scope1/1
  Demux/3 -> Scope2/1
  Demux/1 -> Scope3/1
  Input1/1 -> Demux1/1
  Demux1/1 -> Scope3/2
  Demux1/2 -> Scope1/2
  Demux1/3 -> Scope2/2
  Demux1/4 -> Scope/2
  Demux/4 -> Scope/1

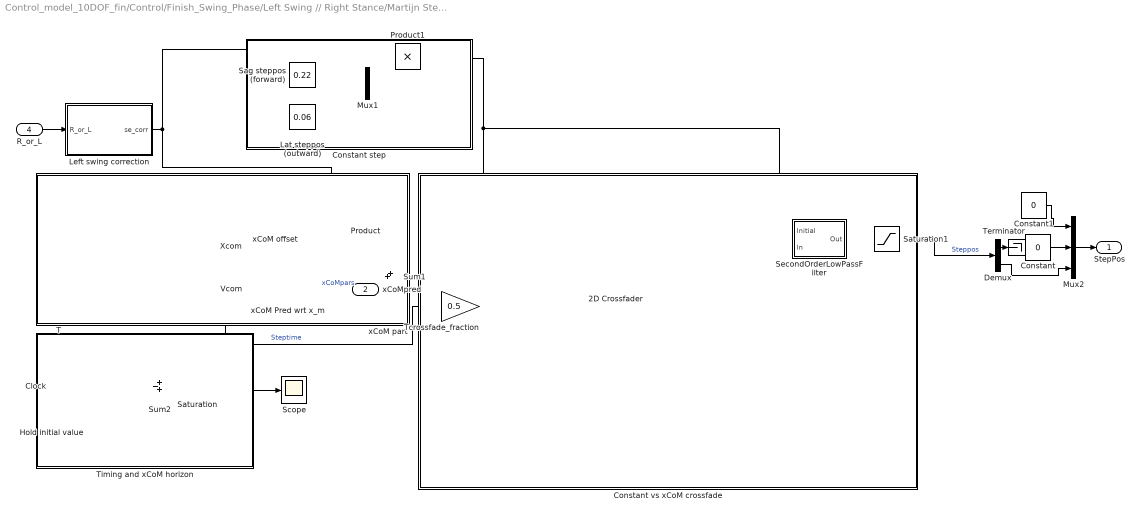
== system Control_model_10DOF_fin/Control/Finish_Swing_Phase/Left Swing // Right Stance/Martijn Step adjustement/xCoM pred ==
  T : Inport
  Xcom : Inport  Port=2
  Vcom : Inport  Port=3
  R_or_L : Inport  Port=4
  2D Crossfader : Subsystem
  Clock : Clock
  Constant : Constant  Value=0
  Constant step : Subsystem
  Constant vs xCoM crossfade : Subsystem
  Constant1 : Constant  Value=0
  Demux : Demux  Outputs=2
  Hold initial value : FootPlacementLibrary/Hold initial value  SystemSampleTime=-1
  Lat steppos (outward) : Constant  Value=0.06
  Left swing correction : Subsystem
  Mux1 : Mux  Inputs=2
  Mux2 : Mux  Inputs=3
  Product : Product
  Product1 : Product
  Sag steppos (forward) : Constant  Value=0.22
  Saturation : Saturate  UpperLimit=0.75  LowerLimit=0
  Saturation1 : Saturate  UpperLimit=[0.3 0.4]  LowerLimit=[-0.3 -0.4]
  Scope : Scope
  SecondOrderLowPassFilter : Subsystem  mask{w=30, z=0.7}
      mask prompts: w "Cut off omega [rad/s]"; z "Zeta"
  Sum1 : Sum  Inputs=++|
  Sum2 : Sum  Inputs=+-+
  Tcrossfade_fraction : Gain  Gain=0.5
  Terminator : Terminator
  Timing and xCoM horizon : Subsystem
  xCoM Pred wrt x_m : Subsystem
  xCoM offset : Constant  Value=[-0.120; 0.03]
  xCoM part : Subsystem
  StepPos : Outport
  xCoMpred : Outport  Port=2
  wires:
  T/1 -> Sum2/1, Tcrossfade_fraction/1  "Steptime"
  Clock/1 -> Sum2/2, Hold initial value/1
  Sum2/1 -> Saturation/1
  Hold initial value/1 -> Sum2/3
  Product/1 -> Sum1/1
  Mux1/1 -> Product1/2
  Sag steppos (forward)/1 -> Mux1/1
  Lat steppos (outward)/1 -> Mux1/2
  Left swing correction/1(se_corr) -> Product1/1, Product/1
  xCoM Pred wrt x_m/1(xCoMpred) -> Sum1/2
  Sum1/1 -> 2D Crossfader/2(xCoM)
  Tcrossfade_fraction/1 -> 2D Crossfader/3(Tcrossfade)
  Saturation/1 -> Scope/1, xCoM Pred wrt x_m/3(trem)
  Product1/1 -> 2D Crossfader/1(ConstStepPos), SecondOrderLowPassFilter/1(Initial)
  2D Crossfader/1(xCoM_crossfaded) -> SecondOrderLowPassFilter/2(In)
  xCoM offset/1 -> Product/2
  Saturation1/1 -> Demux/1  "Steppos"
  SecondOrderLowPassFilter/1(Out) -> Saturation1/1
  Vcom/1 -> xCoM Pred wrt x_m/2(v)
  Xcom/1 -> xCoM Pred wrt x_m/1(x)
  R_or_L/1 -> Left swing correction/1(R_or_L)
  Mux2/1 -> StepPos/1
  Constant/1 -> Mux2/2
  Demux/2 -> Mux2/3
  Constant1/1 -> Mux2/1
  xCoM Pred wrt x_m/2(xCoM pars) -> xCoMpred/1  "xCoMpars"
  Demux/1 -> Terminator/1

== system Control_model_10DOF_fin/Control/Finish_Swing_Phase/Left Swing // Right Stance/Stance leg position_initial/PID right ==
  error : Inport  PortDimensions=4
  velocity : Inport  Port=2
  Integrator : Integrator
  Product : Product  Multiplication=Matrix(*)
  Product2 : Product  Multiplication=Matrix(*)
  Product3 : Product  Multiplication=Matrix(*)
  Sum : Sum  Inputs=++-
  kD : Constant  Value=kD_right
  kI : Constant  Value=kI_right
  kP : Constant  Value=kP_right
  torques_des : Outport  PortDimensions=4  InitialOutput=0
  wires:
  Sum/1 -> torques_des/1
  Product/1 -> Sum/1
  error/1 -> Product2/2, Product/2
  kP/1 -> Product/1
  Integrator/1 -> Sum/2
  Product2/1 -> Integrator/1
  kI/1 -> Product2/1
  kD/1 -> Product3/1
  velocity/1 -> Product3/2
  Product3/1 -> Sum/3

== system Control_model_10DOF_fin/Control/Finish_Swing_Phase/Left Swing // Right Stance/Stance leg position_initial/Scope x2 ==
  Input : Inport
  Input1 : Inport  Port=2
  Demux : Demux
  Demux1 : Demux
  Scope{,1..3} (4 alike) : Scope  NumInputPorts=2
  wires:
  Input/1 -> Demux/1
  Demux/2 -> Scope1/1
  Demux/3 -> Scope2/1
  Demux/1 -> Scope3/1
  Input1/1 -> Demux1/1
  Demux1/1 -> Scope3/2
  Demux1/2 -> Scope1/2
  Demux1/3 -> Scope2/2
  Demux1/4 -> Scope/2
  Demux/4 -> Scope/1

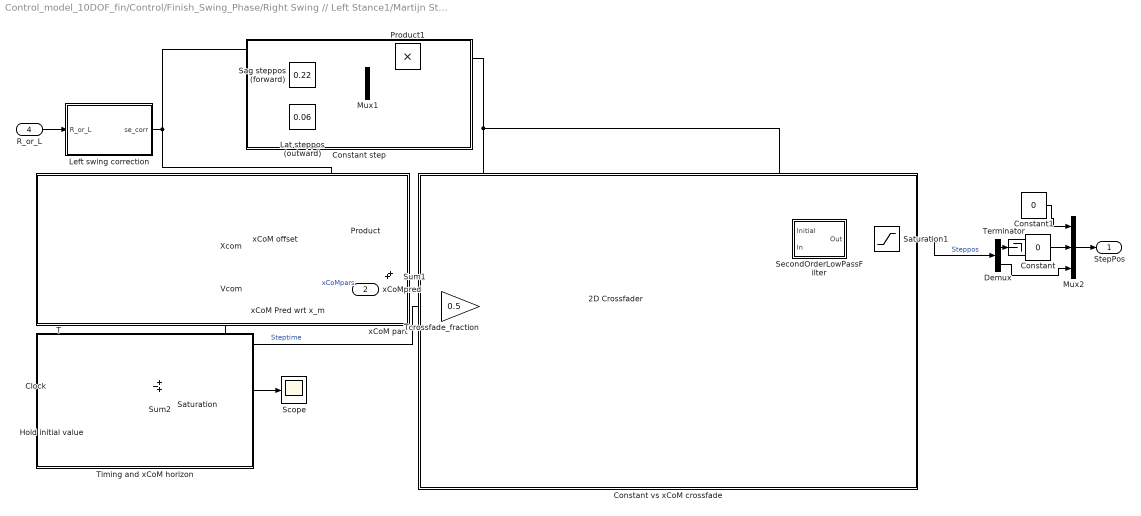
== system Control_model_10DOF_fin/Control/Finish_Swing_Phase/Right Swing // Left Stance1/Martijn Step adjustement/xCoM pred ==
  T : Inport
  Xcom : Inport  Port=2
  Vcom : Inport  Port=3
  R_or_L : Inport  Port=4
  2D Crossfader : Subsystem
  Clock : Clock
  Constant : Constant  Value=0
  Constant step : Subsystem
  Constant vs xCoM crossfade : Subsystem
  Constant1 : Constant  Value=0
  Demux : Demux  Outputs=2
  Hold initial value : FootPlacementLibrary/Hold initial value  SystemSampleTime=-1
  Lat steppos (outward) : Constant  Value=0.06
  Left swing correction : Subsystem
  Mux1 : Mux  Inputs=2
  Mux2 : Mux  Inputs=3
  Product : Product
  Product1 : Product
  Sag steppos (forward) : Constant  Value=0.22
  Saturation : Saturate  UpperLimit=0.75  LowerLimit=0
  Saturation1 : Saturate  UpperLimit=[0.3 0.4]  LowerLimit=[-0.3 -0.4]
  Scope : Scope
  SecondOrderLowPassFilter : Subsystem  mask{w=30, z=0.7}
      mask prompts: w "Cut off omega [rad/s]"; z "Zeta"
  Sum1 : Sum  Inputs=++|
  Sum2 : Sum  Inputs=+-+
  Tcrossfade_fraction : Gain  Gain=0.5
  Terminator : Terminator
  Timing and xCoM horizon : Subsystem
  xCoM Pred wrt x_m : Subsystem
  xCoM offset : Constant  Value=[-0.120; 0.03]
  xCoM part : Subsystem
  StepPos : Outport
  xCoMpred : Outport  Port=2
  wires:
  T/1 -> Sum2/1, Tcrossfade_fraction/1  "Steptime"
  Clock/1 -> Sum2/2, Hold initial value/1
  Sum2/1 -> Saturation/1
  Hold initial value/1 -> Sum2/3
  Product/1 -> Sum1/1
  Mux1/1 -> Product1/2
  Sag steppos (forward)/1 -> Mux1/1
  Lat steppos (outward)/1 -> Mux1/2
  Left swing correction/1(se_corr) -> Product1/1, Product/1
  xCoM Pred wrt x_m/1(xCoMpred) -> Sum1/2
  Sum1/1 -> 2D Crossfader/2(xCoM)
  Tcrossfade_fraction/1 -> 2D Crossfader/3(Tcrossfade)
  Saturation/1 -> Scope/1, xCoM Pred wrt x_m/3(trem)
  Product1/1 -> 2D Crossfader/1(ConstStepPos), SecondOrderLowPassFilter/1(Initial)
  2D Crossfader/1(xCoM_crossfaded) -> SecondOrderLowPassFilter/2(In)
  xCoM offset/1 -> Product/2
  Saturation1/1 -> Demux/1  "Steppos"
  SecondOrderLowPassFilter/1(Out) -> Saturation1/1
  Vcom/1 -> xCoM Pred wrt x_m/2(v)
  Xcom/1 -> xCoM Pred wrt x_m/1(x)
  R_or_L/1 -> Left swing correction/1(R_or_L)
  Mux2/1 -> StepPos/1
  Constant/1 -> Mux2/2
  Demux/2 -> Mux2/3
  Constant1/1 -> Mux2/1
  xCoM Pred wrt x_m/2(xCoM pars) -> xCoMpred/1  "xCoMpars"
  Demux/1 -> Terminator/1

== system Control_model_10DOF_fin/Control/Finish_Swing_Phase/Right Swing // Left Stance1/Right Swing leg control/PID right ==
  error : Inport  PortDimensions=4
  velocity : Inport  Port=2
  Integrator : Integrator
  Product : Product  Multiplication=Matrix(*)
  Product2 : Product  Multiplication=Matrix(*)
  Product3 : Product  Multiplication=Matrix(*)
  Sum : Sum  Inputs=++-
  kD : Constant  Value=kD_right
  kI : Constant  Value=kI_right
  kP : Constant  Value=kP_right
  torques_des : Outport  PortDimensions=4  InitialOutput=0
  wires:
  Sum/1 -> torques_des/1
  Product/1 -> Sum/1
  error/1 -> Product2/2, Product/2
  kP/1 -> Product/1
  Integrator/1 -> Sum/2
  Product2/1 -> Integrator/1
  kI/1 -> Product2/1
  kD/1 -> Product3/1
  velocity/1 -> Product3/2
  Product3/1 -> Sum/3

== system Control_model_10DOF_fin/Control/Finish_Swing_Phase/Right Swing // Left Stance1/Right Swing leg control/Scope x2 ==
  Input : Inport
  Input1 : Inport  Port=2
  Demux : Demux
  Demux1 : Demux
  Gain : Gain  Gain=180/pi
  Gain1 : Gain  Gain=180/pi
  Scope{,1..3} (4 alike) : Scope  NumInputPorts=2
  wires:
  Input/1 -> Gain/1
  Demux/2 -> Scope1/1
  Demux/3 -> Scope2/1
  Demux/1 -> Scope3/1
  Input1/1 -> Gain1/1
  Demux1/1 -> Scope3/2
  Demux1/2 -> Scope1/2
  Demux1/3 -> Scope2/2
  Demux1/4 -> Scope/2
  Demux/4 -> Scope/1
  Gain/1 -> Demux/1
  Gain1/1 -> Demux1/1

== system Control_model_10DOF_fin/Control/Finish_Swing_Phase/Right Swing // Left Stance1/Stance leg position_initial1/PID left ==
  error : Inport  PortDimensions=4
  velocity : Inport  Port=2
  Integrator : Integrator
  Product : Product  Multiplication=Matrix(*)
  Product2 : Product  Multiplication=Matrix(*)
  Product3 : Product  Multiplication=Matrix(*)
  Sum : Sum  Inputs=++-
  kD : Constant  Value=kD_left
  kI : Constant  Value=kI_left
  kP : Constant  Value=kP_left
  torques_des : Outport  PortDimensions=4  InitialOutput=0
  wires:
  Sum/1 -> torques_des/1
  Product/1 -> Sum/1
  error/1 -> Product2/2, Product/2
  kP/1 -> Product/1
  Integrator/1 -> Sum/2
  Product2/1 -> Integrator/1
  kI/1 -> Product2/1
  kD/1 -> Product3/1
  velocity/1 -> Product3/2
  Product3/1 -> Sum/3

== system Control_model_10DOF_fin/Control/Inititial_Transfert/Left stance phase1/Stance leg position_initial/PID right ==
  error : Inport  PortDimensions=4
  velocity : Inport  Port=2
  Integrator : Integrator
  Product : Product  Multiplication=Matrix(*)
  Product2 : Product  Multiplication=Matrix(*)
  Product3 : Product  Multiplication=Matrix(*)
  Sum : Sum  Inputs=++-
  kD : Constant  Value=kD_right
  kI : Constant  Value=kI_right
  kP : Constant  Value=kP_right
  torques_des : Outport  PortDimensions=4  InitialOutput=0
  wires:
  Sum/1 -> torques_des/1
  Product/1 -> Sum/1
  error/1 -> Product2/2, Product/2
  kP/1 -> Product/1
  Integrator/1 -> Sum/2
  Product2/1 -> Integrator/1
  kI/1 -> Product2/1
  kD/1 -> Product3/1
  velocity/1 -> Product3/2
  Product3/1 -> Sum/3

== system Control_model_10DOF_fin/Control/Inititial_Transfert/Left stance phase1/Stance leg position_initial/Scope x1 ==
  Input : Inport
  Demux : Demux
  Scop e1 : Scope
  Scope1 : Scope
  Scope2 : Scope
  Scope3 : Scope
  wires:
  Input/1 -> Demux/1
  Demux/2 -> Scop e1/1
  Demux/3 -> Scope2/1
  Demux/1 -> Scope3/1
  Demux/4 -> Scope1/1

== system Control_model_10DOF_fin/Control/Inititial_Transfert/Left stance phase1/Stance leg position_initial1/PID left ==
  error : Inport  PortDimensions=4
  velocity : Inport  Port=2
  Integrator : Integrator
  Product : Product  Multiplication=Matrix(*)
  Product2 : Product  Multiplication=Matrix(*)
  Product3 : Product  Multiplication=Matrix(*)
  Sum : Sum  Inputs=++-
  kD : Constant  Value=kD_left
  kI : Constant  Value=kI_left
  kP : Constant  Value=kP_left
  torques_des : Outport  PortDimensions=4  InitialOutput=0
  wires:
  Sum/1 -> torques_des/1
  Product/1 -> Sum/1
  error/1 -> Product2/2, Product/2
  kP/1 -> Product/1
  Integrator/1 -> Sum/2
  Product2/1 -> Integrator/1
  kI/1 -> Product2/1
  kD/1 -> Product3/1
  velocity/1 -> Product3/2
  Product3/1 -> Sum/3

== system Control_model_10DOF_fin/Control/Inititial_Transfert/Left stance phase1/Subsystem/Scope x2 ==
  Input : Inport
  Demux : Demux  Outputs=3
  Scope1 : Scope
  Scope2 : Scope
  Scope3 : Scope
  wires:
  Input/1 -> Demux/1
  Demux/2 -> Scope1/1
  Demux/3 -> Scope2/1
  Demux/1 -> Scope3/1

== system Control_model_10DOF_fin/Control/Inititial_Transfert/Left stance phase1/Subsystem/Scope x3 ==
  Input : Inport
  Demux : Demux  Outputs=3
  Scope1 : Scope
  Scope2 : Scope
  Scope3 : Scope
  wires:
  Input/1 -> Demux/1
  Demux/2 -> Scope1/1
  Demux/3 -> Scope2/1
  Demux/1 -> Scope3/1

== system Control_model_10DOF_fin/Control/Inititial_Transfert/Right stance phase/Stance leg position_initial/PID right ==
  error : Inport  PortDimensions=4
  velocity : Inport  Port=2
  Integrator : Integrator
  Product : Product  Multiplication=Matrix(*)
  Product2 : Product  Multiplication=Matrix(*)
  Product3 : Product  Multiplication=Matrix(*)
  Sum : Sum  Inputs=++-
  kD : Constant  Value=kD_right
  kI : Constant  Value=kI_right
  kP : Constant  Value=kP_right
  torques_des : Outport  PortDimensions=4  InitialOutput=0
  wires:
  Sum/1 -> torques_des/1
  Product/1 -> Sum/1
  error/1 -> Product2/2, Product/2
  kP/1 -> Product/1
  Integrator/1 -> Sum/2
  Product2/1 -> Integrator/1
  kI/1 -> Product2/1
  kD/1 -> Product3/1
  velocity/1 -> Product3/2
  Product3/1 -> Sum/3

== system Control_model_10DOF_fin/Control/Inititial_Transfert/Right stance phase/Stance leg position_initial/Scope x2 ==
  Input : Inport
  Input1 : Inport  Port=2
  Demux : Demux
  Demux1 : Demux
  Scope{,1..3} (4 alike) : Scope  NumInputPorts=2
  wires:
  Input/1 -> Demux/1
  Demux/2 -> Scope1/1
  Demux/3 -> Scope2/1
  Demux/1 -> Scope3/1
  Input1/1 -> Demux1/1
  Demux1/1 -> Scope3/2
  Demux1/2 -> Scope1/2
  Demux1/3 -> Scope2/2
  Demux1/4 -> Scope/2
  Demux/4 -> Scope/1

== system Control_model_10DOF_fin/Control/Inititial_Transfert/Right stance phase/Stance leg position_initial1/PID left ==
  error : Inport  PortDimensions=4
  velocity : Inport  Port=2
  Integrator : Integrator
  Product : Product  Multiplication=Matrix(*)
  Product2 : Product  Multiplication=Matrix(*)
  Product3 : Product  Multiplication=Matrix(*)
  Sum : Sum  Inputs=++-
  kD : Constant  Value=kD_left
  kI : Constant  Value=kI_left
  kP : Constant  Value=kP_left
  torques_des : Outport  PortDimensions=4  InitialOutput=0
  wires:
  Sum/1 -> torques_des/1
  Product/1 -> Sum/1
  error/1 -> Product2/2, Product/2
  kP/1 -> Product/1
  Integrator/1 -> Sum/2
  Product2/1 -> Integrator/1
  kI/1 -> Product2/1
  kD/1 -> Product3/1
  velocity/1 -> Product3/2
  Product3/1 -> Sum/3

== system Control_model_10DOF_fin/Control/Inititial_Transfert/Right stance phase/Stance leg position_initial1/Scope x2 ==
  Input : Inport
  Input1 : Inport  Port=2
  Demux : Demux
  Demux1 : Demux
  Scope{,1..3} (4 alike) : Scope  NumInputPorts=2
  wires:
  Input/1 -> Demux/1
  Demux/2 -> Scope1/1
  Demux/3 -> Scope2/1
  Demux/1 -> Scope3/1
  Input1/1 -> Demux1/1
  Demux1/1 -> Scope3/2
  Demux1/2 -> Scope1/2
  Demux1/3 -> Scope2/2
  Demux1/4 -> Scope/2
  Demux/4 -> Scope/1

== system Control_model_10DOF_fin/Control/Single_Support/Left Swing // Right Stance/Left Swing leg control/PID left ==
  error : Inport  PortDimensions=4
  velocity : Inport  Port=2
  Integrator : Integrator
  Product : Product  Multiplication=Matrix(*)
  Product2 : Product  Multiplication=Matrix(*)
  Product3 : Product  Multiplication=Matrix(*)
  Sum : Sum  Inputs=++-
  kD : Constant  Value=kD_left
  kI : Constant  Value=kI_left
  kP : Constant  Value=kP_left
  torques_des : Outport  PortDimensions=4  InitialOutput=0
  wires:
  Sum/1 -> torques_des/1
  Product/1 -> Sum/1
  error/1 -> Product2/2, Product/2
  kP/1 -> Product/1
  Integrator/1 -> Sum/2
  Product2/1 -> Integrator/1
  kI/1 -> Product2/1
  kD/1 -> Product3/1
  velocity/1 -> Product3/2
  Product3/1 -> Sum/3

== system Control_model_10DOF_fin/Control/Single_Support/Left Swing // Right Stance/Left Swing leg control/Scope x1 ==
  Input : Inport
  Demux : Demux  Outputs=3
  Scope1 : Scope
  Scope2 : Scope
  Scope3 : Scope
  wires:
  Input/1 -> Demux/1
  Demux/2 -> Scope1/1
  Demux/3 -> Scope2/1
  Demux/1 -> Scope3/1
